simulink model "UAVIntegratedNavigationSystem"  (R2020b)
settings: Solver=FixedStepAuto  StartTime=0.0  StopTime=TFinal  FixedStep=IMUtime  RelTol=1e-3
values from neighbouring files (symbols this model uses):
  AIONtime = 1    [ModelSettings.m]
  BiasAccel = 9.81E-4    (= 0.000981)    [ModelSettings.m]
  BiasGyro = 2.424068405548E-4    (= 0.000242406840555)    [ModelSettings.m]
  CorrTimeOrientationGNSS = 1    [ModelSettings.m]
  CorrTimePositionGNSS = 1    [ModelSettings.m]
  CorrTimeVelocityGNSS = 1    [ModelSettings.m]
  delay = 1.5    [ModelSettings.m]
  e = 0.081819106    [ModelSettings.m]
  g0 = 9.780327    [ModelSettings.m]
  GNSStime = 0.2    [ModelSettings.m]
  H0 = 0.1    [ModelSettings.m]
  IMUtime = 0.01    [ModelSettings.m]
  indUAV = 2    [ModelSettings.m]
  LambdaInit = 0.6555    [ModelSettings.m]
  mass = 0.7    [ModelSettings.m]
  N = 100    [ModelSettings.m]
  PhiInit = 0.968    [ModelSettings.m]
  PitchDown = -PitchUp    (= -0.1)    [ModelSettings.m]
  PitchUp = 0.1    [ModelSettings.m]
  Ra = 6378.245    [ModelSettings.m]
  RollDown = -RollUp    (= -0.1)    [ModelSettings.m]
  RollUp = 0.1    [ModelSettings.m]
  SigmaAccel = 9.81E-4    (= 0.000981)    [ModelSettings.m]
  SigmaAION = 30    [ModelSettings.m]
  SigmaAltitudeGNSS = 3    [ModelSettings.m]
  SigmaGyro = 2.666475246102E-6    (= 2.6664752461e-06)    [ModelSettings.m]
  SigmaLaser = 5    [ModelSettings.m]
  SigmaOrientationGNSS = 0.00349    [ModelSettings.m]
  SigmaPositionGNSS = 1.5    [ModelSettings.m]
  SigmaVelocityGNSS = 0.03    [ModelSettings.m]
  SigmaVelocityUpGNSS = 0.03    [ModelSettings.m]
  U1down = 0    [ModelSettings.m]
  U1up = 4 * ForceCoeff * OmegaMax^2    (= 9.9858124)    [ModelSettings.m]
  U2down = -U2up    (= -2.4964531)    [ModelSettings.m]
  U2up = ForceCoeff * OmegaMax^2    (= 2.4964531)    [ModelSettings.m]
  U3down = -U3up    (= -2.4964531)    [ModelSettings.m]
  U3up = ForceCoeff * OmegaMax^2    (= 2.4964531)    [ModelSettings.m]
  U4down = -U4up    (= -0.2494604)    [ModelSettings.m]
  U4up = 2 * DragCoeff * OmegaMax^2    (= 0.2494604)    [ModelSettings.m]
  WEarth = 7.2921158553E-5    (= 7.2921158553e-05)    [ModelSettings.m]
undefined symbols (not defined in the file or in its folder): deg, Newton, rad, Raphson, s
libraries: simulink x11, sharedtransform x7, pid_lib x6, aerolibconvert2 x4, sharedutil x4
(part 3 of 5)

== system UAVIntegratedNavigationSystem/Subsystem1/Функционирование приемника ГНСС/If Action Subsystem4 ==
  Action Port : ActionPort  ActionPortLabel=if(u1 == -1)
  Bus Creator : BusCreator  Inputs=3
  Mux1 : Mux  Inputs=3
  Mux2 : Mux  Inputs=3
  Mux3 : Mux  Inputs=3
  NaN{,1..8} (9 alike) : Constant  Value=NaN  OutDataTypeStr=Inherit: Inherit via back propagation
  Out1 : Outport
  wires:
  NaN5/1 -> Mux2/3  "<VelZ>"
  NaN1/1 -> Mux1/2  "<Y>"
  NaN4/1 -> Mux2/2  "<VelY>"
  Mux1/1 -> Bus Creator/1
  NaN3/1 -> Mux2/1  "<VelX>"
  NaN/1 -> Mux1/1  "<X>"
  Mux2/1 -> Bus Creator/2
  NaN6/1 -> Mux3/1  "<Roll>"
  NaN2/1 -> Mux1/3  "<Z>"
  Mux3/1 -> Bus Creator/3
  NaN8/1 -> Mux3/2  "<Psi>"
  NaN7/1 -> Mux3/3  "<Pitch>"
  Bus Creator/1 -> Out1/1

== system UAVIntegratedNavigationSystem/Subsystem1/Функционирование приемника ГНСС/If Action Subsystem5 ==
  In1 : Inport
  Action Port : ActionPort  ActionPortLabel=else
  Out1 : Outport
  wires:
  In1/1 -> Out1/1

== system UAVIntegratedNavigationSystem/Алгоритм ИНС /Алгоритм Навигации/Координаты БПЛА (Географ. СК) ==
  Velocity : Inport
  R : Inport  Port=2
  "Север(0), Восток(0)" : Inport  Port=3
  Demux : Demux  Outputs=2
  Demux1 : Demux  Outputs=3
  Demux2 : Demux  Outputs=2
  Integrator : Integrator  InitialCondition=PhiInit
  Integrator1 : Integrator  InitialConditionSource=external
  Integrator2 : Integrator
  Integrator3 : Integrator  InitialConditionSource=external
  Mux : Mux
  Terminator : Terminator
  dPhi/dt : Product  Inputs=*/
  "Coord, phi" : Outport
  wires:
  R/1 -> Demux/1
  dPhi/dt/1 -> Integrator/1
  Demux/1 -> dPhi/dt/2
  Velocity/1 -> Demux1/1
  Demux1/1 -> dPhi/dt/1, Integrator1/1
  Mux/1 -> "Coord, phi"/1
  Demux/2 -> Terminator/1
  Integrator1/1 -> Mux/1
  Integrator2/1 -> Mux/2
  Integrator3/1 -> Mux/3
  Demux1/2 -> Integrator2/1
  Demux1/3 -> Integrator3/1
  Integrator/1 -> Mux/4
  "Север(0), Восток(0)"/1 -> Demux2/1
  Demux2/1 -> Integrator1/2
  Demux2/2 -> Integrator3/2

== system UAVIntegratedNavigationSystem/Алгоритм ИНС /Алгоритм Навигации/Радиус - вектор точки местоположения Ц.М. БПЛА (phi) ==
  Phi : Inport
  Add2 : Sum  Inputs=+-
  Add3 : Sum  Inputs=+-
  Add4 : Sum
  Add5 : Sum
  Constant2 : Constant  Value=Ra
  Constant3 : Constant  Value=H0
  Constant4 : Constant
  Constant5 : Constant  Value=1.5
  Divide : Product  Inputs=*/
  Divide1 : Product  Inputs=*/
  Mux : Mux  Inputs=2
  Power : Math  Operator=pow  SaturateOnIntegerOverflow=on
  Product1 : Product
  Product2 : Product
  Sin1 : Trigonometry
  Sqrt : Sqrt  SaturateOnIntegerOverflow=on
  Square2 : Math  Operator=square  SaturateOnIntegerOverflow=on
  Square3 : Math  Operator=square  SaturateOnIntegerOverflow=on
  e1 : Constant  Value=e
  "km -> m" : Gain  Gain=1000
  "km -> m 1" : Gain  Gain=1000
  "R, м" : Outport
  wires:
  Phi/1 -> Sin1/1
  Constant2/1 -> "km -> m"/1
  Constant3/1 -> "km -> m 1"/1
  e1/1 -> Square2/1
  Square2/1 -> Product2/1, Add2/2
  Constant4/1 -> Add2/1, Add3/1
  "km -> m"/1 -> Product1/1, Divide1/1
  Add2/1 -> Product1/2
  Sin1/1 -> Square3/1
  Square3/1 -> Product2/2
  Product2/1 -> Add3/2
  Product1/1 -> Divide/1
  Divide/1 -> Add4/1
  "km -> m 1"/1 -> Add5/1, Add4/2
  Add4/1 -> Mux/1  "R1"
  Add3/1 -> Power/1, Sqrt/1
  Power/1 -> Divide/2
  Constant5/1 -> Power/2
  Mux/1 -> "R, м"/1
  Sqrt/1 -> Divide1/2
  Divide1/1 -> Add5/2
  Add5/1 -> Mux/2  "R2"

== system UAVIntegratedNavigationSystem/Алгоритм ИНС /Алгоритм Навигации/Скорости БПЛА (Географ. СК) ==
  AccX : Inport
  AccY : Inport  Port=2
  AccZ : Inport  Port=3
  R : Inport  Port=4
  phi : Inport  Port=5
  Integrator : Integrator
  Integrator1 : Integrator
  Integrator2 : Integrator
  Mux : Mux  Inputs=3
  dVx / dt : Subsystem
  dVy / dt : Subsystem
  dVz / dt : Subsystem
  Velocity : Outport
  wires:
  Integrator/1 -> dVz / dt/5(Vx), dVy / dt/4(Vx), dVx / dt/5(Vx), Mux/1
  Integrator1/1 -> dVz / dt/3(Vy), dVx / dt/3(Vy), Mux/2
  Integrator2/1 -> Mux/3, dVz / dt/4(Vz), dVx / dt/4(Vz), dVy / dt/3(Vz)
  AccX/1 -> dVx / dt/1(AccX)
  R/1 -> dVz / dt/2(R), dVy / dt/2(R), dVx / dt/2(R)
  dVx / dt/1(dVx/dt) -> Integrator/1
  AccY/1 -> dVy / dt/1(AccY)
  dVy / dt/1(dVy/dt) -> Integrator1/1
  AccZ/1 -> dVz / dt/1(AccZ)
  dVz / dt/1(dVz/dt) -> Integrator2/1
  Mux/1 -> Velocity/1
  phi/1 -> dVx / dt/6(phi), dVy / dt/5(phi), dVz / dt/6(phi)

== system UAVIntegratedNavigationSystem/Алгоритм ИНС /Алгоритм Навигации/Угловая скорость вращения трехгранника ==
  Velocity : Inport
  R : Inport  Port=2
  phi : Inport  Port=3
  Add : Sum
  Constant : Constant  Value=0
  Cos : Trigonometry  Operator=cos
  Demux2 : Demux  Outputs=3
  Demux3 : Demux  Outputs=2
  Divide : Product  Inputs=*/
  Divide1 : Product  Inputs=*/
  Divide2 : Product  Inputs=*/
  Gain : Gain  Gain=-1
  Mux : Mux  Inputs=3
  Mux1 : Mux  Inputs=3
  Sin : Trigonometry
  Terminator3 : Terminator
  WEarth : Gain  Gain=WEarth
  WEarth1 : Gain  Gain=WEarth
  OmegaG : Outport
  wires:
  Demux2/3 -> Divide/1, Divide1/1
  phi/1 -> Sin/1, Cos/1
  WEarth1/1 -> Mux1/2
  Cos/1 -> WEarth/1
  Divide/1 -> Mux/1
  Sin/1 -> WEarth1/1
  WEarth/1 -> Mux1/1
  R/1 -> Demux3/1
  Constant/1 -> Mux1/3
  Demux3/2 -> Divide1/2
  Mux/1 -> Add/2
  Demux2/1 -> Gain/1
  Add/1 -> OmegaG/1
  Demux2/2 -> Terminator3/1
  Demux3/1 -> Divide/2, Divide2/2
  Divide2/1 -> Mux/3
  Divide1/1 -> Mux/2
  Mux1/1 -> Add/1
  Gain/1 -> Divide2/1
  Velocity/1 -> Demux2/1

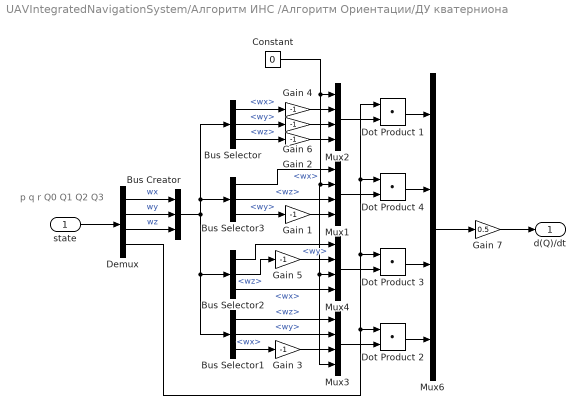
== system UAVIntegratedNavigationSystem/Алгоритм ИНС /Алгоритм Ориентации/ДУ кватерниона ==
  note: p q r Q0 Q1 Q2 Q3
  state : Inport
  Bus Creator : BusCreator  Inputs=3
  Bus Selector : BusSelector  OutputSignals=wx,wy,wz
  Bus Selector1 : BusSelector  OutputSignals=wz,wy,wx
  Bus Selector2 : BusSelector  OutputSignals=wy,wz,wx
  Bus Selector3 : BusSelector  OutputSignals=wx,wz,wy
  Constant : Constant  Value=0
  Demux : Demux  Outputs=[1 1 1 4]
      settings: DisplayOption=none
  Dot Product {1..4} (4 alike) : DotProduct  InputSameDT=on  OutDataTypeStr=Inherit: Inherit via internal rule
  Gain {1..6} (6 alike) : Gain  Gain=-1  SaturateOnIntegerOverflow=on  OutDataTypeStr=Inherit: Same as input  ParamDataTypeStr=Inherit: Same as input
  Gain 7 : Gain  Gain=0.5  SaturateOnIntegerOverflow=on  OutDataTypeStr=Inherit: Same as input  ParamDataTypeStr=Inherit: Same as input
  Mux{1..4,6} (5 alike) : Mux
  d(Q)/dt : Outport
  wires:
  Mux6/1 -> Gain 7/1
  state/1 -> Demux/1
  Gain 2/1 -> Mux2/4
  Bus Selector/1 -> Gain 4/1  "<wx>"
  Mux2/1 -> Dot Product 1/2
  Mux3/1 -> Dot Product 2/2
  Mux4/1 -> Dot Product 3/2
  Demux/1 -> Bus Creator/1  "wx"
  Demux/2 -> Bus Creator/2  "wy"
  Demux/3 -> Bus Creator/3  "wz"
  Gain 5/1 -> Mux4/2
  Gain 3/1 -> Mux3/3
  Mux1/1 -> Dot Product 4/2
  Bus Creator/1 -> Bus Selector2/1, Bus Selector1/1, Bus Selector/1, Bus Selector3/1
  Constant/1 -> Mux2/1, Mux1/2, Mux3/4, Mux4/3
  Bus Selector3/3 -> Gain 1/1  "<wy>"
  Gain 4/1 -> Mux2/2
  Gain 6/1 -> Mux2/3
  Bus Selector/2 -> Gain 6/1  "<wy>"
  Bus Selector/3 -> Gain 2/1  "<wz>"
  Dot Product 2/1 -> Mux6/4
  Dot Product 3/1 -> Mux6/3
  Dot Product 4/1 -> Mux6/2
  Dot Product 1/1 -> Mux6/1
  Demux/4 -> Dot Product 3/1, Dot Product 4/1, Dot Product 1/1, Dot Product 2/1
  Gain 7/1 -> d(Q)/dt/1
  Bus Selector3/1 -> Mux1/1  "<wx>"
  Bus Selector3/2 -> Mux1/3  "<wz>"
  Gain 1/1 -> Mux1/4
  Bus Selector1/3 -> Gain 3/1  "<wx>"
  Bus Selector1/2 -> Mux3/2  "<wy>"
  Bus Selector1/1 -> Mux3/1  "<wz>"
  Bus Selector2/1 -> Mux4/1  "<wy>"
  Bus Selector2/2 -> Gain 5/1  "<wz>"
  Bus Selector2/3 -> Mux4/4  "<wx>"

== system UAVIntegratedNavigationSystem/Алгоритм ИНС /Алгоритм Ориентации/Нормирование кватерниона ==
  q : Inport  PortDimensions=4
  Product : Product  Inputs=*/  InputSameDT=on  RndMeth=Zero  SaturateOnIntegerOverflow=on  OutDataTypeStr=Inherit: Same as first input
  Square : Math  Operator=square  SignedPower=on  SaturateOnIntegerOverflow=on
  Square Root : Sqrt  Operator=signedSqrt  AlgorithmType=Newton-Raphson  SaturateOnIntegerOverflow=on
  Sum : Sum  Inputs=1  InputSameDT=on  SaturateOnIntegerOverflow=on  OutDataTypeStr=Inherit: Same as first input
  qnorm : Outport  PortDimensions=4
  wires:
  Product/1 -> qnorm/1
  Square Root/1 -> Product/2
  Square/1 -> Sum/1
  Sum/1 -> Square Root/1
  q/1 -> Product/1, Square/1

== system UAVIntegratedNavigationSystem/Алгоритм ИНС (коррекия БЧЭ)/Алгоритм Навигации/Координаты БПЛА (Географ. СК) ==
  Velocity : Inport
  R : Inport  Port=2
  "Север(0), Восток(0)" : Inport  Port=3
  Demux : Demux  Outputs=2
  Demux1 : Demux  Outputs=3
  Demux2 : Demux  Outputs=2
  Integrator : Integrator  InitialCondition=PhiInit
  Integrator1 : Integrator  InitialConditionSource=external
  Integrator2 : Integrator
  Integrator3 : Integrator  InitialConditionSource=external
  Mux : Mux
  Terminator : Terminator
  dPhi/dt : Product  Inputs=*/
  "Coord, phi" : Outport
  wires:
  R/1 -> Demux/1
  dPhi/dt/1 -> Integrator/1
  Demux/1 -> dPhi/dt/2
  Velocity/1 -> Demux1/1
  Demux1/1 -> dPhi/dt/1, Integrator1/1
  Mux/1 -> "Coord, phi"/1
  Demux/2 -> Terminator/1
  Integrator1/1 -> Mux/1
  Integrator2/1 -> Mux/2
  Integrator3/1 -> Mux/3
  Demux1/2 -> Integrator2/1
  Demux1/3 -> Integrator3/1
  Integrator/1 -> Mux/4
  "Север(0), Восток(0)"/1 -> Demux2/1
  Demux2/1 -> Integrator1/2
  Demux2/2 -> Integrator3/2

== system UAVIntegratedNavigationSystem/Алгоритм ИНС (коррекия БЧЭ)/Алгоритм Навигации/Радиус - вектор точки местоположения Ц.М. БПЛА (phi) ==
  Phi : Inport
  Add2 : Sum  Inputs=+-
  Add3 : Sum  Inputs=+-
  Add4 : Sum
  Add5 : Sum
  Constant2 : Constant  Value=Ra
  Constant3 : Constant  Value=H0
  Constant4 : Constant
  Constant5 : Constant  Value=1.5
  Divide : Product  Inputs=*/
  Divide1 : Product  Inputs=*/
  Mux : Mux  Inputs=2
  Power : Math  Operator=pow  SaturateOnIntegerOverflow=on
  Product1 : Product
  Product2 : Product
  Sin1 : Trigonometry
  Sqrt : Sqrt  SaturateOnIntegerOverflow=on
  Square2 : Math  Operator=square  SaturateOnIntegerOverflow=on
  Square3 : Math  Operator=square  SaturateOnIntegerOverflow=on
  e1 : Constant  Value=e
  "km -> m" : Gain  Gain=1000
  "km -> m 1" : Gain  Gain=1000
  "R, м" : Outport
  wires:
  Phi/1 -> Sin1/1
  Constant2/1 -> "km -> m"/1
  Constant3/1 -> "km -> m 1"/1
  e1/1 -> Square2/1
  Square2/1 -> Product2/1, Add2/2
  Constant4/1 -> Add2/1, Add3/1
  "km -> m"/1 -> Product1/1, Divide1/1
  Add2/1 -> Product1/2
  Sin1/1 -> Square3/1
  Square3/1 -> Product2/2
  Product2/1 -> Add3/2
  Product1/1 -> Divide/1
  Divide/1 -> Add4/1
  "km -> m 1"/1 -> Add5/1, Add4/2
  Add4/1 -> Mux/1  "R1"
  Add3/1 -> Power/1, Sqrt/1
  Power/1 -> Divide/2
  Constant5/1 -> Power/2
  Mux/1 -> "R, м"/1
  Sqrt/1 -> Divide1/2
  Divide1/1 -> Add5/2
  Add5/1 -> Mux/2  "R2"

== system UAVIntegratedNavigationSystem/Алгоритм ИНС (коррекия БЧЭ)/Алгоритм Навигации/Скорости БПЛА (Географ. СК) ==
  AccX : Inport
  AccY : Inport  Port=2
  AccZ : Inport  Port=3
  R : Inport  Port=4
  phi : Inport  Port=5
  Integrator : Integrator
  Integrator1 : Integrator
  Integrator2 : Integrator
  Mux : Mux  Inputs=3
  dVx / dt : Subsystem
  dVy / dt : Subsystem
  dVz / dt : Subsystem
  Velocity : Outport
  wires:
  Integrator/1 -> dVz / dt/5(Vx), dVy / dt/4(Vx), dVx / dt/5(Vx), Mux/1
  Integrator1/1 -> dVz / dt/3(Vy), dVx / dt/3(Vy), Mux/2
  Integrator2/1 -> Mux/3, dVz / dt/4(Vz), dVx / dt/4(Vz), dVy / dt/3(Vz)
  AccX/1 -> dVx / dt/1(AccX)
  R/1 -> dVz / dt/2(R), dVy / dt/2(R), dVx / dt/2(R)
  dVx / dt/1(dVx/dt) -> Integrator/1
  AccY/1 -> dVy / dt/1(AccY)
  dVy / dt/1(dVy/dt) -> Integrator1/1
  AccZ/1 -> dVz / dt/1(AccZ)
  dVz / dt/1(dVz/dt) -> Integrator2/1
  Mux/1 -> Velocity/1
  phi/1 -> dVx / dt/6(phi), dVy / dt/5(phi), dVz / dt/6(phi)

== system UAVIntegratedNavigationSystem/Алгоритм ИНС (коррекия БЧЭ)/Алгоритм Навигации/Угловая скорость вращения трехгранника ==
  Velocity : Inport
  R : Inport  Port=2
  phi : Inport  Port=3
  Add : Sum
  Constant : Constant  Value=0
  Cos : Trigonometry  Operator=cos
  Demux2 : Demux  Outputs=3
  Demux3 : Demux  Outputs=2
  Divide : Product  Inputs=*/
  Divide1 : Product  Inputs=*/
  Divide2 : Product  Inputs=*/
  Gain : Gain  Gain=-1
  Mux : Mux  Inputs=3
  Mux1 : Mux  Inputs=3
  Sin : Trigonometry
  Terminator3 : Terminator
  WEarth : Gain  Gain=WEarth
  WEarth1 : Gain  Gain=WEarth
  OmegaG : Outport
  wires:
  Demux2/3 -> Divide/1, Divide1/1
  phi/1 -> Sin/1, Cos/1
  WEarth1/1 -> Mux1/2
  Cos/1 -> WEarth/1
  Divide/1 -> Mux/1
  Sin/1 -> WEarth1/1
  WEarth/1 -> Mux1/1
  R/1 -> Demux3/1
  Constant/1 -> Mux1/3
  Demux3/2 -> Divide1/2
  Mux/1 -> Add/2
  Demux2/1 -> Gain/1
  Add/1 -> OmegaG/1
  Demux2/2 -> Terminator3/1
  Demux3/1 -> Divide/2, Divide2/2
  Divide2/1 -> Mux/3
  Divide1/1 -> Mux/2
  Mux1/1 -> Add/1
  Gain/1 -> Divide2/1
  Velocity/1 -> Demux2/1

== system UAVIntegratedNavigationSystem/Алгоритм ИНС (коррекия БЧЭ)/Алгоритм Ориентации/ДУ кватерниона ==
  note: p q r Q0 Q1 Q2 Q3
  state : Inport
  Bus Creator : BusCreator  Inputs=3
  Bus Selector : BusSelector  OutputSignals=wx,wy,wz
  Bus Selector1 : BusSelector  OutputSignals=wz,wy,wx
  Bus Selector2 : BusSelector  OutputSignals=wy,wz,wx
  Bus Selector3 : BusSelector  OutputSignals=wx,wz,wy
  Constant : Constant  Value=0
  Demux : Demux  Outputs=[1 1 1 4]
      settings: DisplayOption=none
  Dot Product {1..4} (4 alike) : DotProduct  InputSameDT=on  OutDataTypeStr=Inherit: Inherit via internal rule
  Gain {1..6} (6 alike) : Gain  Gain=-1  SaturateOnIntegerOverflow=on  OutDataTypeStr=Inherit: Same as input  ParamDataTypeStr=Inherit: Same as input
  Gain 7 : Gain  Gain=0.5  SaturateOnIntegerOverflow=on  OutDataTypeStr=Inherit: Same as input  ParamDataTypeStr=Inherit: Same as input
  Mux{1..4,6} (5 alike) : Mux
  d(Q)/dt : Outport
  wires:
  Mux6/1 -> Gain 7/1
  state/1 -> Demux/1
  Gain 2/1 -> Mux2/4
  Bus Selector/1 -> Gain 4/1  "<wx>"
  Mux2/1 -> Dot Product 1/2
  Mux3/1 -> Dot Product 2/2
  Mux4/1 -> Dot Product 3/2
  Demux/1 -> Bus Creator/1  "wx"
  Demux/2 -> Bus Creator/2  "wy"
  Demux/3 -> Bus Creator/3  "wz"
  Gain 5/1 -> Mux4/2
  Gain 3/1 -> Mux3/3
  Mux1/1 -> Dot Product 4/2
  Bus Creator/1 -> Bus Selector2/1, Bus Selector1/1, Bus Selector/1, Bus Selector3/1
  Constant/1 -> Mux2/1, Mux1/2, Mux3/4, Mux4/3
  Bus Selector3/3 -> Gain 1/1  "<wy>"
  Gain 4/1 -> Mux2/2
  Gain 6/1 -> Mux2/3
  Bus Selector/2 -> Gain 6/1  "<wy>"
  Bus Selector/3 -> Gain 2/1  "<wz>"
  Dot Product 2/1 -> Mux6/4
  Dot Product 3/1 -> Mux6/3
  Dot Product 4/1 -> Mux6/2
  Dot Product 1/1 -> Mux6/1
  Demux/4 -> Dot Product 3/1, Dot Product 4/1, Dot Product 1/1, Dot Product 2/1
  Gain 7/1 -> d(Q)/dt/1
  Bus Selector3/1 -> Mux1/1  "<wx>"
  Bus Selector3/2 -> Mux1/3  "<wz>"
  Gain 1/1 -> Mux1/4
  Bus Selector1/3 -> Gain 3/1  "<wx>"
  Bus Selector1/2 -> Mux3/2  "<wy>"
  Bus Selector1/1 -> Mux3/1  "<wz>"
  Bus Selector2/1 -> Mux4/1  "<wy>"
  Bus Selector2/2 -> Gain 5/1  "<wz>"
  Bus Selector2/3 -> Mux4/4  "<wx>"

== system UAVIntegratedNavigationSystem/Алгоритм ИНС (коррекия БЧЭ)/Алгоритм Ориентации/Нормирование кватерниона ==
  q : Inport  PortDimensions=4
  Product : Product  Inputs=*/  InputSameDT=on  RndMeth=Zero  SaturateOnIntegerOverflow=on  OutDataTypeStr=Inherit: Same as first input
  Square : Math  Operator=square  SignedPower=on  SaturateOnIntegerOverflow=on
  Square Root : Sqrt  Operator=signedSqrt  AlgorithmType=Newton-Raphson  SaturateOnIntegerOverflow=on
  Sum : Sum  Inputs=1  InputSameDT=on  SaturateOnIntegerOverflow=on  OutDataTypeStr=Inherit: Same as first input
  qnorm : Outport  PortDimensions=4
  wires:
  Product/1 -> qnorm/1
  Square Root/1 -> Product/2
  Square/1 -> Sum/1
  Sum/1 -> Square Root/1
  q/1 -> Product/1, Square/1

== system UAVIntegratedNavigationSystem/Блок модели динамики квадрокоптера + САУ/Полетный контроллер/Ограничение управляющих сил ==
  U1* : Inport
  U2* : Inport  Port=2
  U3* : Inport  Port=3
  U4* : Inport  Port=4
  Limit U1 : Saturate  UpperLimit=U1up  LowerLimit=U1down
  Limit U2 : Saturate  UpperLimit=U2up  LowerLimit=U2down
  Limit U3 : Saturate  UpperLimit=U3up  LowerLimit=U3down
  Limit U4 : Saturate  UpperLimit=U4up  LowerLimit=U4down
  U1 : Outport
  U2 : Outport  Port=2
  U3 : Outport  Port=3
  U4 : Outport  Port=4
  wires:
  Limit U2/1 -> U2/1
  U2*/1 -> Limit U2/1
  U1*/1 -> Limit U1/1
  Limit U1/1 -> U1/1
  U4*/1 -> Limit U4/1
  Limit U4/1 -> U4/1
  Limit U3/1 -> U3/1
  U3*/1 -> Limit U3/1

== system UAVIntegratedNavigationSystem/Блок модели динамики квадрокоптера + САУ/Полетный контроллер/Угловая стабилизация ==
  Roll* : Inport
  Roll : Inport  Port=2
  Pitch* : Inport  Port=3
  Pitch : Inport  Port=4
  Psi* : Inport  Port=5
  Psi : Inport  Port=6
  RollPID : Inport  Port=7
  PitchPID : Inport  Port=8
  PsiPID : Inport  Port=9
  Constant : Constant  Value=N
  Demux : Demux  Outputs=3
  Demux1 : Demux  Outputs=3
  Demux2 : Demux  Outputs=3
  PID Pitch : pid_lib/PID Controller  Controller=PID  Form=Parallel  TimeDomain=Continuous-time  UseExternalTs=off  SampleTime=-1  IntegratorMethod=Forward Euler  FilterMethod=Forward Euler  ControllerParametersSource=external  P=1  I=0  D=0  UseFilter=on  N=100  TunerSelectOption=Transfer Function Based (PID Tuner App)  InitialConditionSource=internal  InitialConditionForIntegrator=0  InitialConditionForFilter=0  DifferentiatorICPrevScaledInput=0  ExternalReset=none  TrackingMode=off  Kt=1  LimitOutput=off  SatLimitsSource=internal  UpperSaturationLimit=inf  LowerSaturationLimit=-inf  LinearizeAsGain=on  AntiWindupMode=none  Kb=1  POutMin=[]  POutMax=[]  IOutMin=[]  IOutMax=[]  DOutMin=[]  DOutMax=[]  NOutMin=[]  NOutMax=[]  SumOutMin=[]  SumOutMax=[]  SaturationOutMin=[]  SaturationOutMax=[]  PParamMin=[]  PParamMax=[]  IParamMin=[]  IParamMax=[]  DParamMin=[]  DParamMax=[]  NParamMin=[]  NParamMax=[]  KbParamMin=[]  KbParamMax=[]  KtParamMin=[]  KtParamMax=[]  KbOutMin=[]  KbOutMax=[]  KtOutMin=[]  KtOutMax=[]  IntegratorOutMin=[]  IntegratorOutMax=[]  FilterOutMin=[]  FilterOutMax=[]  SumI1OutMin=[]  SumI1OutMax=[]  SumI2OutMin=[]  SumI2OutMax=[]  SumI3OutMin=[]  SumI3OutMax=[]  SumI4OutMin=[]  SumI4OutMax=[]  SumDOutMin=[]  SumDOutMax=[]  DifferentiatorOutMin=[]  DifferentiatorOutMax=[]  FilterDiffOutCoefMin=[]  FilterDiffOutCoefMax=[]  ReciprocalOutMin=[]  ReciprocalOutMax=[]  SumDenOutMin=[]  SumDenOutMax=[]  SumNumOutMin=[]  SumNumOutMax=[]  DivideOutMin=[]  DivideOutMax=[]  UdiffTsProdOutMin=[]  UdiffTsProdOutMax=[]  NTsProdOutMin=[]  NTsProdOutMax=[]  UintegralTsProdOutMin=[]  UintegralTsProdOutMax=[]  UngainTsProdOutMin=[]  UngainTsProdOutMax=[]  IntegratorContinuousStateAttributes=''  IntegratorStateMustResolveToSignalObject=off  IntegratorRTWStateStorageClass=Auto  FilterContinuousStateAttributes=''  FilterStateMustResolveToSignalObject=off  FilterRTWStateStorageClass=Auto  ParallelPVariant=ExternalParameters  IdealPVariant=Disabled  IVariant=ExternalParameters  DVariant=ExternalParameters  IntegratorVariant=Continuous  SatVariant=Disabled  AWVariant=Passthrough  PCopyVariant=Disabled  TRVariant=Disabled  FdbkBlocksVariant=Forward  IdealPFdbkVariant=Disabled  SatFdbkVariant=Disabled  DerivativeFilterVariant=ContFilter  NVariant=ExternalParameters  NCopyVariant=Disabled  FilterICVariant=InternalICsFilter  IntegratorICVariant=InternalICs  ExternalResetVariant=Disabled  TRSumVariant=Passthrough  SumFdbkVariant=Disabled  SumVariant=Sum_PID  TsampFilterVariant=InternalTs  TsampNgainVariant=Passthrough  TsampIntegralVariant=Passthrough  ExternalSaturationOutDataTypeStr=Inherit: Same as second input
  PID Psi : pid_lib/PID Controller  Controller=PID  Form=Parallel  TimeDomain=Continuous-time  UseExternalTs=off  SampleTime=-1  IntegratorMethod=Forward Euler  FilterMethod=Forward Euler  ControllerParametersSource=external  P=1  I=0  D=0  UseFilter=on  N=100  TunerSelectOption=Transfer Function Based (PID Tuner App)  InitialConditionSource=internal  InitialConditionForIntegrator=0  InitialConditionForFilter=0  DifferentiatorICPrevScaledInput=0  ExternalReset=none  TrackingMode=off  Kt=1  LimitOutput=off  SatLimitsSource=internal  UpperSaturationLimit=inf  LowerSaturationLimit=-inf  LinearizeAsGain=on  AntiWindupMode=none  Kb=1  POutMin=[]  POutMax=[]  IOutMin=[]  IOutMax=[]  DOutMin=[]  DOutMax=[]  NOutMin=[]  NOutMax=[]  SumOutMin=[]  SumOutMax=[]  SaturationOutMin=[]  SaturationOutMax=[]  PParamMin=[]  PParamMax=[]  IParamMin=[]  IParamMax=[]  DParamMin=[]  DParamMax=[]  NParamMin=[]  NParamMax=[]  KbParamMin=[]  KbParamMax=[]  KtParamMin=[]  KtParamMax=[]  KbOutMin=[]  KbOutMax=[]  KtOutMin=[]  KtOutMax=[]  IntegratorOutMin=[]  IntegratorOutMax=[]  FilterOutMin=[]  FilterOutMax=[]  SumI1OutMin=[]  SumI1OutMax=[]  SumI2OutMin=[]  SumI2OutMax=[]  SumI3OutMin=[]  SumI3OutMax=[]  SumI4OutMin=[]  SumI4OutMax=[]  SumDOutMin=[]  SumDOutMax=[]  DifferentiatorOutMin=[]  DifferentiatorOutMax=[]  FilterDiffOutCoefMin=[]  FilterDiffOutCoefMax=[]  ReciprocalOutMin=[]  ReciprocalOutMax=[]  SumDenOutMin=[]  SumDenOutMax=[]  SumNumOutMin=[]  SumNumOutMax=[]  DivideOutMin=[]  DivideOutMax=[]  UdiffTsProdOutMin=[]  UdiffTsProdOutMax=[]  NTsProdOutMin=[]  NTsProdOutMax=[]  UintegralTsProdOutMin=[]  UintegralTsProdOutMax=[]  UngainTsProdOutMin=[]  UngainTsProdOutMax=[]  IntegratorContinuousStateAttributes=''  IntegratorStateMustResolveToSignalObject=off  IntegratorRTWStateStorageClass=Auto  FilterContinuousStateAttributes=''  FilterStateMustResolveToSignalObject=off  FilterRTWStateStorageClass=Auto  ParallelPVariant=ExternalParameters  IdealPVariant=Disabled  IVariant=ExternalParameters  DVariant=ExternalParameters  IntegratorVariant=Continuous  SatVariant=Disabled  AWVariant=Passthrough  PCopyVariant=Disabled  TRVariant=Disabled  FdbkBlocksVariant=Forward  IdealPFdbkVariant=Disabled  SatFdbkVariant=Disabled  DerivativeFilterVariant=ContFilter  NVariant=ExternalParameters  NCopyVariant=Disabled  FilterICVariant=InternalICsFilter  IntegratorICVariant=InternalICs  ExternalResetVariant=Disabled  TRSumVariant=Passthrough  SumFdbkVariant=Disabled  SumVariant=Sum_PID  TsampFilterVariant=InternalTs  TsampNgainVariant=Passthrough  TsampIntegralVariant=Passthrough  ExternalSaturationOutDataTypeStr=Inherit: Same as second input
  PID Roll : pid_lib/PID Controller  Controller=PID  Form=Parallel  TimeDomain=Continuous-time  UseExternalTs=off  SampleTime=-1  IntegratorMethod=Forward Euler  FilterMethod=Forward Euler  ControllerParametersSource=external  P=1  I=0  D=0  UseFilter=on  N=100  TunerSelectOption=Transfer Function Based (PID Tuner App)  InitialConditionSource=internal  InitialConditionForIntegrator=0  InitialConditionForFilter=0  DifferentiatorICPrevScaledInput=0  ExternalReset=none  TrackingMode=off  Kt=1  LimitOutput=off  SatLimitsSource=internal  UpperSaturationLimit=inf  LowerSaturationLimit=-inf  LinearizeAsGain=on  AntiWindupMode=none  Kb=1  POutMin=[]  POutMax=[]  IOutMin=[]  IOutMax=[]  DOutMin=[]  DOutMax=[]  NOutMin=[]  NOutMax=[]  SumOutMin=[]  SumOutMax=[]  SaturationOutMin=[]  SaturationOutMax=[]  PParamMin=[]  PParamMax=[]  IParamMin=[]  IParamMax=[]  DParamMin=[]  DParamMax=[]  NParamMin=[]  NParamMax=[]  KbParamMin=[]  KbParamMax=[]  KtParamMin=[]  KtParamMax=[]  KbOutMin=[]  KbOutMax=[]  KtOutMin=[]  KtOutMax=[]  IntegratorOutMin=[]  IntegratorOutMax=[]  FilterOutMin=[]  FilterOutMax=[]  SumI1OutMin=[]  SumI1OutMax=[]  SumI2OutMin=[]  SumI2OutMax=[]  SumI3OutMin=[]  SumI3OutMax=[]  SumI4OutMin=[]  SumI4OutMax=[]  SumDOutMin=[]  SumDOutMax=[]  DifferentiatorOutMin=[]  DifferentiatorOutMax=[]  FilterDiffOutCoefMin=[]  FilterDiffOutCoefMax=[]  ReciprocalOutMin=[]  ReciprocalOutMax=[]  SumDenOutMin=[]  SumDenOutMax=[]  SumNumOutMin=[]  SumNumOutMax=[]  DivideOutMin=[]  DivideOutMax=[]  UdiffTsProdOutMin=[]  UdiffTsProdOutMax=[]  NTsProdOutMin=[]  NTsProdOutMax=[]  UintegralTsProdOutMin=[]  UintegralTsProdOutMax=[]  UngainTsProdOutMin=[]  UngainTsProdOutMax=[]  IntegratorContinuousStateAttributes=''  IntegratorStateMustResolveToSignalObject=off  IntegratorRTWStateStorageClass=Auto  FilterContinuousStateAttributes=''  FilterStateMustResolveToSignalObject=off  FilterRTWStateStorageClass=Auto  ParallelPVariant=ExternalParameters  IdealPVariant=Disabled  IVariant=ExternalParameters  DVariant=ExternalParameters  IntegratorVariant=Continuous  SatVariant=Disabled  AWVariant=Passthrough  PCopyVariant=Disabled  TRVariant=Disabled  FdbkBlocksVariant=Forward  IdealPFdbkVariant=Disabled  SatFdbkVariant=Disabled  DerivativeFilterVariant=ContFilter  NVariant=ExternalParameters  NCopyVariant=Disabled  FilterICVariant=InternalICsFilter  IntegratorICVariant=InternalICs  ExternalResetVariant=Disabled  TRSumVariant=Passthrough  SumFdbkVariant=Disabled  SumVariant=Sum_PID  TsampFilterVariant=InternalTs  TsampNgainVariant=Passthrough  TsampIntegralVariant=Passthrough  ExternalSaturationOutDataTypeStr=Inherit: Same as second input
  Sum1 : Sum  Inputs=|+-
  Sum3 : Sum  Inputs=|+-
  Sum4 : Sum  Inputs=|+-
  U2* : Outport
  U3* : Outport  Port=2
  U4* : Outport  Port=3
  wires:
  Pitch/1 -> Sum4/2
  Psi*/1 -> Sum3/1
  PID Psi/1 -> U4*/1
  Roll/1 -> Sum1/2
  PID Pitch/1 -> U3*/1
  Roll*/1 -> Sum1/1
  Psi/1 -> Sum3/2
  PID Roll/1 -> U2*/1
  Pitch*/1 -> Sum4/1
  Sum1/1 -> PID Roll/1
  Sum4/1 -> PID Pitch/1
  Sum3/1 -> PID Psi/1
  RollPID/1 -> Demux/1
  Demux/3 -> PID Roll/4
  Demux/1 -> PID Roll/2
  Demux/2 -> PID Roll/3
  Constant/1 -> PID Psi/5, PID Pitch/5, PID Roll/5
  Demux1/1 -> PID Pitch/2
  Demux1/2 -> PID Pitch/3
  Demux1/3 -> PID Pitch/4
  PitchPID/1 -> Demux1/1
  Demux2/1 -> PID Psi/2
  Demux2/2 -> PID Psi/3
  Demux2/3 -> PID Psi/4
  PsiPID/1 -> Demux2/1

== system UAVIntegratedNavigationSystem/Блок модели динамики квадрокоптера + САУ/Полетный контроллер/Удержание высоты  ==
  Y* : Inport
  Y : Inport  Port=2
  g : Inport  Port=3
  AltPID : Inport  Port=4
  Add : Sum
  Constant : Constant  Value=N
  Demux : Demux  Outputs=3
  PID Altitude : pid_lib/PID Controller  Controller=PID  Form=Parallel  TimeDomain=Continuous-time  UseExternalTs=off  SampleTime=-1  IntegratorMethod=Forward Euler  FilterMethod=Forward Euler  ControllerParametersSource=external  P=1  I=0  D=0  UseFilter=on  N=100  TunerSelectOption=Transfer Function Based (PID Tuner App)  InitialConditionSource=internal  InitialConditionForIntegrator=0  InitialConditionForFilter=0  DifferentiatorICPrevScaledInput=0  ExternalReset=none  TrackingMode=off  Kt=1  LimitOutput=off  SatLimitsSource=internal  UpperSaturationLimit=inf  LowerSaturationLimit=-inf  LinearizeAsGain=on  AntiWindupMode=none  Kb=1  POutMin=[]  POutMax=[]  IOutMin=[]  IOutMax=[]  DOutMin=[]  DOutMax=[]  NOutMin=[]  NOutMax=[]  SumOutMin=[]  SumOutMax=[]  SaturationOutMin=[]  SaturationOutMax=[]  PParamMin=[]  PParamMax=[]  IParamMin=[]  IParamMax=[]  DParamMin=[]  DParamMax=[]  NParamMin=[]  NParamMax=[]  KbParamMin=[]  KbParamMax=[]  KtParamMin=[]  KtParamMax=[]  KbOutMin=[]  KbOutMax=[]  KtOutMin=[]  KtOutMax=[]  IntegratorOutMin=[]  IntegratorOutMax=[]  FilterOutMin=[]  FilterOutMax=[]  SumI1OutMin=[]  SumI1OutMax=[]  SumI2OutMin=[]  SumI2OutMax=[]  SumI3OutMin=[]  SumI3OutMax=[]  SumI4OutMin=[]  SumI4OutMax=[]  SumDOutMin=[]  SumDOutMax=[]  DifferentiatorOutMin=[]  DifferentiatorOutMax=[]  FilterDiffOutCoefMin=[]  FilterDiffOutCoefMax=[]  ReciprocalOutMin=[]  ReciprocalOutMax=[]  SumDenOutMin=[]  SumDenOutMax=[]  SumNumOutMin=[]  SumNumOutMax=[]  DivideOutMin=[]  DivideOutMax=[]  UdiffTsProdOutMin=[]  UdiffTsProdOutMax=[]  NTsProdOutMin=[]  NTsProdOutMax=[]  UintegralTsProdOutMin=[]  UintegralTsProdOutMax=[]  UngainTsProdOutMin=[]  UngainTsProdOutMax=[]  IntegratorContinuousStateAttributes=''  IntegratorStateMustResolveToSignalObject=off  IntegratorRTWStateStorageClass=Auto  FilterContinuousStateAttributes=''  FilterStateMustResolveToSignalObject=off  FilterRTWStateStorageClass=Auto  ParallelPVariant=ExternalParameters  IdealPVariant=Disabled  IVariant=ExternalParameters  DVariant=ExternalParameters  IntegratorVariant=Continuous  SatVariant=Disabled  AWVariant=Passthrough  PCopyVariant=Disabled  TRVariant=Disabled  FdbkBlocksVariant=Forward  IdealPFdbkVariant=Disabled  SatFdbkVariant=Disabled  DerivativeFilterVariant=ContFilter  NVariant=ExternalParameters  NCopyVariant=Disabled  FilterICVariant=InternalICsFilter  IntegratorICVariant=InternalICs  ExternalResetVariant=Disabled  TRSumVariant=Passthrough  SumFdbkVariant=Disabled  SumVariant=Sum_PID  TsampFilterVariant=InternalTs  TsampNgainVariant=Passthrough  TsampIntegralVariant=Passthrough  ExternalSaturationOutDataTypeStr=Inherit: Same as second input
  Sum : Sum  Inputs=|+-
  mass : Gain  Gain=mass
  U1* : Outport
  wires:
  Y*/1 -> Sum/1
  Y/1 -> Sum/2
  Add/1 -> U1*/1
  mass/1 -> Add/2
  Sum/1 -> PID Altitude/1
  PID Altitude/1 -> Add/1
  g/1 -> mass/1
  AltPID/1 -> Demux/1
  Demux/1 -> PID Altitude/2
  Demux/2 -> PID Altitude/3
  Demux/3 -> PID Altitude/4
  Constant/1 -> PID Altitude/5

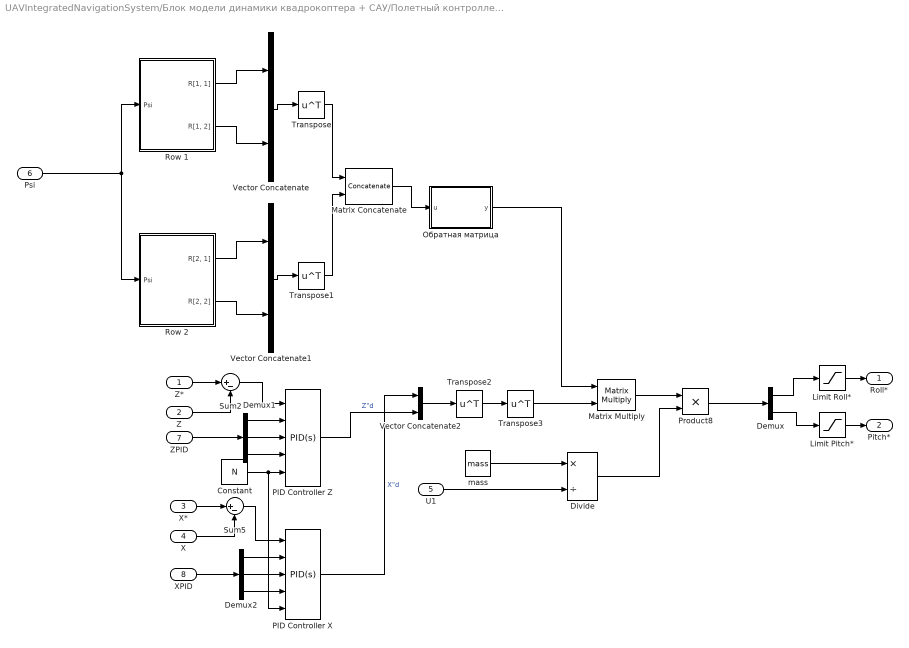
== system UAVIntegratedNavigationSystem/Блок модели динамики квадрокоптера + САУ/Полетный контроллер/Удержание положения ==
  Z* : Inport
  Z : Inport  Port=2
  X* : Inport  Port=3
  X : Inport  Port=4
  U1 : Inport  Port=5
  Psi : Inport  Port=6
  ZPID : Inport  Port=7
  XPID : Inport  Port=8
  Constant : Constant  Value=N
  Demux : Demux  Outputs=2
  Demux1 : Demux  Outputs=3
  Demux2 : Demux  Outputs=3
  Divide : Product  Inputs=*/
  Limit Pitch* : Saturate  UpperLimit=PitchUp  LowerLimit=PitchDown
  Limit Roll* : Saturate  UpperLimit=RollUp  LowerLimit=RollDown
  Matrix Concatenate : Concatenate  Mode=Multidimensional array
  Matrix Multiply : Product  Multiplication=Matrix(*)
  PID Controller X : pid_lib/PID Controller  Controller=PID  Form=Parallel  TimeDomain=Continuous-time  UseExternalTs=off  SampleTime=-1  IntegratorMethod=Forward Euler  FilterMethod=Forward Euler  ControllerParametersSource=external  P=1  I=0  D=0  UseFilter=on  N=100  TunerSelectOption=Transfer Function Based (PID Tuner App)  InitialConditionSource=internal  InitialConditionForIntegrator=0  InitialConditionForFilter=0  DifferentiatorICPrevScaledInput=0  ExternalReset=none  TrackingMode=off  Kt=1  LimitOutput=off  SatLimitsSource=internal  UpperSaturationLimit=inf  LowerSaturationLimit=-inf  LinearizeAsGain=on  AntiWindupMode=none  Kb=1  POutMin=[]  POutMax=[]  IOutMin=[]  IOutMax=[]  DOutMin=[]  DOutMax=[]  NOutMin=[]  NOutMax=[]  SumOutMin=[]  SumOutMax=[]  SaturationOutMin=[]  SaturationOutMax=[]  PParamMin=[]  PParamMax=[]  IParamMin=[]  IParamMax=[]  DParamMin=[]  DParamMax=[]  NParamMin=[]  NParamMax=[]  KbParamMin=[]  KbParamMax=[]  KtParamMin=[]  KtParamMax=[]  KbOutMin=[]  KbOutMax=[]  KtOutMin=[]  KtOutMax=[]  IntegratorOutMin=[]  IntegratorOutMax=[]  FilterOutMin=[]  FilterOutMax=[]  SumI1OutMin=[]  SumI1OutMax=[]  SumI2OutMin=[]  SumI2OutMax=[]  SumI3OutMin=[]  SumI3OutMax=[]  SumI4OutMin=[]  SumI4OutMax=[]  SumDOutMin=[]  SumDOutMax=[]  DifferentiatorOutMin=[]  DifferentiatorOutMax=[]  FilterDiffOutCoefMin=[]  FilterDiffOutCoefMax=[]  ReciprocalOutMin=[]  ReciprocalOutMax=[]  SumDenOutMin=[]  SumDenOutMax=[]  SumNumOutMin=[]  SumNumOutMax=[]  DivideOutMin=[]  DivideOutMax=[]  UdiffTsProdOutMin=[]  UdiffTsProdOutMax=[]  NTsProdOutMin=[]  NTsProdOutMax=[]  UintegralTsProdOutMin=[]  UintegralTsProdOutMax=[]  UngainTsProdOutMin=[]  UngainTsProdOutMax=[]  IntegratorContinuousStateAttributes=''  IntegratorStateMustResolveToSignalObject=off  IntegratorRTWStateStorageClass=Auto  FilterContinuousStateAttributes=''  FilterStateMustResolveToSignalObject=off  FilterRTWStateStorageClass=Auto  ParallelPVariant=ExternalParameters  IdealPVariant=Disabled  IVariant=ExternalParameters  DVariant=ExternalParameters  IntegratorVariant=Continuous  SatVariant=Disabled  AWVariant=Passthrough  PCopyVariant=Disabled  TRVariant=Disabled  FdbkBlocksVariant=Forward  IdealPFdbkVariant=Disabled  SatFdbkVariant=Disabled  DerivativeFilterVariant=ContFilter  NVariant=ExternalParameters  NCopyVariant=Disabled  FilterICVariant=InternalICsFilter  IntegratorICVariant=InternalICs  ExternalResetVariant=Disabled  TRSumVariant=Passthrough  SumFdbkVariant=Disabled  SumVariant=Sum_PID  TsampFilterVariant=InternalTs  TsampNgainVariant=Passthrough  TsampIntegralVariant=Passthrough  ExternalSaturationOutDataTypeStr=Inherit: Same as second input
  PID Controller Z : pid_lib/PID Controller  Controller=PID  Form=Parallel  TimeDomain=Continuous-time  UseExternalTs=off  SampleTime=-1  IntegratorMethod=Forward Euler  FilterMethod=Forward Euler  ControllerParametersSource=external  P=1  I=0  D=0  UseFilter=on  N=100  TunerSelectOption=Transfer Function Based (PID Tuner App)  InitialConditionSource=internal  InitialConditionForIntegrator=0  InitialConditionForFilter=0  DifferentiatorICPrevScaledInput=0  ExternalReset=none  TrackingMode=off  Kt=1  LimitOutput=off  SatLimitsSource=internal  UpperSaturationLimit=inf  LowerSaturationLimit=-inf  LinearizeAsGain=on  AntiWindupMode=none  Kb=1  POutMin=[]  POutMax=[]  IOutMin=[]  IOutMax=[]  DOutMin=[]  DOutMax=[]  NOutMin=[]  NOutMax=[]  SumOutMin=[]  SumOutMax=[]  SaturationOutMin=[]  SaturationOutMax=[]  PParamMin=[]  PParamMax=[]  IParamMin=[]  IParamMax=[]  DParamMin=[]  DParamMax=[]  NParamMin=[]  NParamMax=[]  KbParamMin=[]  KbParamMax=[]  KtParamMin=[]  KtParamMax=[]  KbOutMin=[]  KbOutMax=[]  KtOutMin=[]  KtOutMax=[]  IntegratorOutMin=[]  IntegratorOutMax=[]  FilterOutMin=[]  FilterOutMax=[]  SumI1OutMin=[]  SumI1OutMax=[]  SumI2OutMin=[]  SumI2OutMax=[]  SumI3OutMin=[]  SumI3OutMax=[]  SumI4OutMin=[]  SumI4OutMax=[]  SumDOutMin=[]  SumDOutMax=[]  DifferentiatorOutMin=[]  DifferentiatorOutMax=[]  FilterDiffOutCoefMin=[]  FilterDiffOutCoefMax=[]  ReciprocalOutMin=[]  ReciprocalOutMax=[]  SumDenOutMin=[]  SumDenOutMax=[]  SumNumOutMin=[]  SumNumOutMax=[]  DivideOutMin=[]  DivideOutMax=[]  UdiffTsProdOutMin=[]  UdiffTsProdOutMax=[]  NTsProdOutMin=[]  NTsProdOutMax=[]  UintegralTsProdOutMin=[]  UintegralTsProdOutMax=[]  UngainTsProdOutMin=[]  UngainTsProdOutMax=[]  IntegratorContinuousStateAttributes=''  IntegratorStateMustResolveToSignalObject=off  IntegratorRTWStateStorageClass=Auto  FilterContinuousStateAttributes=''  FilterStateMustResolveToSignalObject=off  FilterRTWStateStorageClass=Auto  ParallelPVariant=ExternalParameters  IdealPVariant=Disabled  IVariant=ExternalParameters  DVariant=ExternalParameters  IntegratorVariant=Continuous  SatVariant=Disabled  AWVariant=Passthrough  PCopyVariant=Disabled  TRVariant=Disabled  FdbkBlocksVariant=Forward  IdealPFdbkVariant=Disabled  SatFdbkVariant=Disabled  DerivativeFilterVariant=ContFilter  NVariant=ExternalParameters  NCopyVariant=Disabled  FilterICVariant=InternalICsFilter  IntegratorICVariant=InternalICs  ExternalResetVariant=Disabled  TRSumVariant=Passthrough  SumFdbkVariant=Disabled  SumVariant=Sum_PID  TsampFilterVariant=InternalTs  TsampNgainVariant=Passthrough  TsampIntegralVariant=Passthrough  ExternalSaturationOutDataTypeStr=Inherit: Same as second input
  Product8 : Product
  Row 1 : Subsystem
  Row 2 : Subsystem
  Sum2 : Sum  Inputs=|+-
  Sum5 : Sum  Inputs=|+-
  Transpose{,1..3} (4 alike) : Math  Operator=transpose  SaturateOnIntegerOverflow=on
  Vector Concatenate : Concatenate
  Vector Concatenate1 : Concatenate
  Vector Concatenate2 : Concatenate
  mass : Constant  Value=mass
  "Обратная матрица " : MATLAB Function  TreatAsAtomicUnit=on
  Roll* : Outport
  Pitch* : Outport  Port=2
  wires:
  Z*/1 -> Sum2/1
  X*/1 -> Sum5/1
  Z/1 -> Sum2/2
  Sum2/1 -> PID Controller Z/1
  Sum5/1 -> PID Controller X/1
  X/1 -> Sum5/2
  U1/1 -> Divide/2
  mass/1 -> Divide/1
  Psi/1 -> Row 1/1(Psi), Row 2/1(Psi)
  PID Controller Z/1 -> Vector Concatenate2/2  "Z\"d"
  Divide/1 -> Product8/2
  PID Controller X/1 -> Vector Concatenate2/1  "X\"d"
  Transpose1/1 -> Matrix Concatenate/2
  Transpose/1 -> Matrix Concatenate/1
  Vector Concatenate/1 -> Transpose/1
  Row 2/2("R[2, 2]") -> Vector Concatenate1/2
  Vector Concatenate1/1 -> Transpose1/1
  Row 1/2("R[1, 2]") -> Vector Concatenate/2
  Row 2/1("R[2, 1]") -> Vector Concatenate1/1
  Row 1/1("R[1, 1]") -> Vector Concatenate/1
  Matrix Concatenate/1 -> "Обратная матрица "/1(u)
  "Обратная матрица "/1(y) -> Matrix Multiply/1
  Vector Concatenate2/1 -> Transpose2/1
  Transpose2/1 -> Transpose3/1
  Transpose3/1 -> Matrix Multiply/2
  Matrix Multiply/1 -> Product8/1
  Product8/1 -> Demux/1
  Demux/2 -> Limit Pitch*/1
  Demux/1 -> Limit Roll*/1
  Limit Roll*/1 -> Roll*/1
  Limit Pitch*/1 -> Pitch*/1
  Constant/1 -> PID Controller X/5, PID Controller Z/5
  ZPID/1 -> Demux1/1
  Demux1/1 -> PID Controller Z/2
  Demux1/2 -> PID Controller Z/3
  Demux1/3 -> PID Controller Z/4
  Demux2/1 -> PID Controller X/2
  Demux2/2 -> PID Controller X/3
  Demux2/3 -> PID Controller X/4
  XPID/1 -> Demux2/1

== system UAVIntegratedNavigationSystem/Блок модели динамики квадрокоптера + САУ/Упрощенная динамика БЛА /Векторы ускорений действующих сил ==
  U1 : Inport
  Pitch : Inport  Port=2
  Roll : Inport  Port=3
  Psi : Inport  Port=4
  g : Inport  Port=5
  "(X, Y, Z, phi)" : Inport  Port=6
  Относительное и Кориолисово ускорение : Inport  Port=7
  Bus Creator : BusCreator  Inputs=4
  Demux : Demux  Outputs=2
  Gain : Gain  Gain=-1
  Ускорение силы гравитации : Subsystem
  Ускорение силы тяги : Subsystem
  "Векторы ускорений, 3 x [3 x 1]" : Outport
  wires:
  Ускорение силы гравитации/1(Вектор ускорения силы гравитации) -> Bus Creator/2  "Вектор ускорения силы гравитации [3 x 1]"
  Ускорение силы тяги/1(Вектор ускорения силы тяги) -> Bus Creator/1  "Вектор ускорения силы тяги [3 x 1]"
  Roll/1 -> Ускорение силы тяги/3(Roll)
  U1/1 -> Ускорение силы тяги/1(U1)
  Pitch/1 -> Ускорение силы тяги/2(Pitch)
  Psi/1 -> Ускорение силы тяги/4(Psi)
  g/1 -> Ускорение силы гравитации/1(g)
  Bus Creator/1 -> "Векторы ускорений, 3 x [3 x 1]"/1
  "(X, Y, Z, phi)"/1 -> Ускорение силы гравитации/2("(X, Y, Z, phi)")
  Относительное и Кориолисово ускорение/1 -> Gain/1
  Demux/1 -> Bus Creator/3  "Вектор относительного ускорения [3 x 1]"
  Gain/1 -> Demux/1
  Demux/2 -> Bus Creator/4  "Вектор Кориолисова ускорения [3 x 1]"

== system UAVIntegratedNavigationSystem/Блок модели динамики квадрокоптера + САУ/Упрощенная динамика БЛА /Моменты управляемых сил ==
  U2 : Inport
  U4 : Inport  Port=2
  U3 : Inport  Port=3
  Mux : Mux  Inputs=3
  "(Mx,My, Mz)" : Outport
  wires:
  U4/1 -> Mux/2
  Mux/1 -> "(Mx,My, Mz)"/1
  U2/1 -> Mux/1
  U3/1 -> Mux/3

== system UAVIntegratedNavigationSystem/Блок модели динамики квадрокоптера + САУ/Упрощенная динамика БЛА /Простр. движение Ц.М. БПЛА (Геогр. СК) ==
  Acc X : Inport
  Acc Y : Inport  Port=2
  AccZ : Inport  Port=3
  "Север(0), Восток(0)" : Inport  Port=4
  Bus Selector : BusSelector  OutputSignals=phi
  Demux1 : Demux  Outputs=3
  Demux2 : Demux  Outputs=2
  Divide : Product  Inputs=*/
  Divide1 : Product  Inputs=*/
  Divide2 : Product  Inputs=*/
  Gain : Gain  Gain=-1
  Mux : Mux  Inputs=3
  Terminator3 : Terminator
  Координаты БПЛА (Географ. СК) : Subsystem
  Радиус - вектор точки местоположения Ц.М. БПЛА (phi) : Subsystem
  Скорости БПЛА (Географ. СК) : Subsystem
  "(X, Y, Z, phi, lambda)" : Outport
  (Vx,Vy,Vz) : Outport  Port=2
  Относительное и Кориолисово ускорение : Outport  Port=3
  Угловая скорость вращения трехгранника : Outport  Port=4
  wires:
  Радиус - вектор точки местоположения Ц.М. БПЛА (phi)/1("R, м") -> Demux2/1, Координаты БПЛА (Географ. СК)/2(R), Скорости БПЛА (Географ. СК)/4(R)
  Скорости БПЛА (Географ. СК)/1(Velocity) -> (Vx,Vy,Vz)/1, Demux1/1, Координаты БПЛА (Географ. СК)/1(Velocity)
  Acc Y/1 -> Скорости БПЛА (Географ. СК)/2(AccY)
  Координаты БПЛА (Географ. СК)/1("Coord, phi, lambda") -> "(X, Y, Z, phi, lambda)"/1, Bus Selector/1
  Acc X/1 -> Скорости БПЛА (Географ. СК)/1(AccX)
  AccZ/1 -> Скорости БПЛА (Географ. СК)/3(AccZ)
  Bus Selector/1 -> Радиус - вектор точки местоположения Ц.М. БПЛА (phi)/1(Phi), Скорости БПЛА (Географ. СК)/5(phi)  "<phi>"
  Скорости БПЛА (Географ. СК)/2(Относ и Кориолис ускорение) -> Относительное и Кориолисово ускорение/1
  Mux/1 -> Угловая скорость вращения трехгранника/1
  Divide/1 -> Mux/1
  Demux1/3 -> Divide1/1, Divide/1
  Demux2/1 -> Divide/2, Divide2/2
  Divide1/1 -> Mux/2
  Demux2/2 -> Divide1/2
  Demux1/2 -> Terminator3/1
  Divide2/1 -> Mux/3
  Demux1/1 -> Gain/1
  Gain/1 -> Divide2/1
  "Север(0), Восток(0)"/1 -> Координаты БПЛА (Географ. СК)/3("Север(0), Восток(0)")

== system UAVIntegratedNavigationSystem/Блок модели динамики квадрокоптера + САУ/Упрощенная динамика БЛА /Решение уравнения Пуассона ==
  AngVelocity : Inport
  Demux : Demux  Outputs=3
  Integrator : Integrator  InitialCondition=[1, 0, 0, 0]
  Mux4 : Mux  Inputs=2
  Quaternions to Rotation Angles : sharedtransform/Quaternions to Rotation Angles  rotationOrder=YZX  aMode=aMode
      settings: SourceProductBaseCode=AE,PW,MT,UV,VE,VP
  ДУ кватернион : Subsystem
  Нормирование кватерниона : Subsystem
  Roll : Outport
  Pitch : Outport  Port=2
  Psi : Outport  Port=3
  wires:
  Integrator/1 -> Нормирование кватерниона/1(q)
  ДУ кватернион/1(d(Q)/dt) -> Integrator/1
  Нормирование кватерниона/1(qnorm) -> Quaternions to Rotation Angles/1, Mux4/2
  Mux4/1 -> ДУ кватернион/1(state)  "Wx Wy Wz  Q0-Q3"
  Quaternions to Rotation Angles/1 -> Demux/1
  Demux/1 -> Psi/1  "Psi"
  Demux/3 -> Roll/1  "Roll"
  Demux/2 -> Pitch/1  "Pitch"
  AngVelocity/1 -> Mux4/1

== system UAVIntegratedNavigationSystem/Показания АИОН + ЛД/Измерения АИОН + ЛД/Вектор случайных аддитивных ошибок в определении высоты местоположения БЛА ==
  "ФФ " : Subsystem
  Вектор измерительных шумов [1x1] : Outport
  wires:
  "ФФ "/1(Случ. погрешность ЛД по высоте) -> Вектор измерительных шумов [1x1]/1

== system UAVIntegratedNavigationSystem/Показания АИОН + ЛД/Измерения АИОН + ЛД/Вектор случайных аддитивных ошибок в определении координат местоположения БЛА ==
  Mux1 : Mux  Inputs=2
  "ФФ " : Subsystem
  Вектор измерительных шумов [2x1] : Outport
  wires:
  Mux1/1 -> Вектор измерительных шумов [2x1]/1
  "ФФ "/1(Случ. погрешность АИОНпо координатам) -> Mux1/2, Mux1/1

== system UAVIntegratedNavigationSystem/Показания приемника ГНСС/Измерения ГНСС/Вектор случайных аддитивных ошибок в определении координат местопложения БЛА ==
  Mux1 : Mux  Inputs=3
  "ФФ " : Subsystem
  ФФ 1 : Subsystem
  Вектор измерительных шумов [3x1] : Outport
  wires:
  Mux1/1 -> Вектор измерительных шумов [3x1]/1
  "ФФ "/1(Случ. погрешность ГНСС по координатам) -> Mux1/3, Mux1/1
  ФФ 1/1(Случ. погрешность ГНСС по высоте) -> Mux1/2

== system UAVIntegratedNavigationSystem/Показания приемника ГНСС/Измерения ГНСС/Вектор случайных аддитивных ошибок в определении ориентации БЛА ==
  Mux1 : Mux  Inputs=3
  "ФФ " : Subsystem
  Вектор измерительных шумов [3x1] : Outport
  wires:
  Mux1/1 -> Вектор измерительных шумов [3x1]/1
  "ФФ "/1(Случ. погрешность ГНСС по углам) -> Mux1/2, Mux1/3, Mux1/1

== system UAVIntegratedNavigationSystem/Показания приемника ГНСС/Измерения ГНСС/Вектор случайных аддитивных ошибок в определении проекций скорости  БЛА ==
  Mux1 : Mux  Inputs=3
  "ФФ " : Subsystem
  ФФ 1 : Subsystem
  Вектор измерительных шумов [3x1] : Outport
  wires:
  "ФФ "/1(Случ. погрешность ГНСС по скоростям) -> Mux1/3, Mux1/1
  Mux1/1 -> Вектор измерительных шумов [3x1]/1
  ФФ 1/1(Случ. погрешность ГНСС по скоростям) -> Mux1/2

== system UAVIntegratedNavigationSystem/Алгоритм ИНС /Алгоритм Навигации/Скорости БПЛА (Географ. СК)/dVx // dt ==
  AccX : Inport
  R : Inport  Port=2
  Vy : Inport  Port=3
  Vz : Inport  Port=4
  Vx : Inport  Port=5
  phi : Inport  Port=6
  AccX Кориолис : Subsystem
  AccX Относительное : Subsystem
  Add : Sum  Inputs=+++
  dVx/dt : Outport
  wires:
  AccX/1 -> Add/1
  Add/1 -> dVx/dt/1
  R/1 -> AccX Относительное/4(R)
  Vx/1 -> AccX Относительное/1(VelX)
  Vy/1 -> AccX Относительное/2(VelY)
  Vz/1 -> AccX Кориолис/1(VelZ), AccX Относительное/3(VelZ)
  phi/1 -> AccX Кориолис/2(phi), AccX Относительное/5(phi)
  AccX Относительное/1(AccX Относительное) -> Add/2
  AccX Кориолис/1(AccX Кориолис) -> Add/3

== system UAVIntegratedNavigationSystem/Алгоритм ИНС /Алгоритм Навигации/Скорости БПЛА (Географ. СК)/dVy // dt ==
  AccY : Inport
  R : Inport  Port=2
  Vz : Inport  Port=3
  Vx : Inport  Port=4
  phi : Inport  Port=5
  AccY Кориолис : Subsystem
  AccY Относительное : Subsystem
  Add : Sum  Inputs=+++
  dVy/dt : Outport
  wires:
  AccY/1 -> Add/1
  Vx/1 -> AccY Относительное/1(VelX)
  R/1 -> AccY Относительное/3(R)
  Add/1 -> dVy/dt/1
  Vz/1 -> AccY Кориолис/1(VelZ), AccY Относительное/2(VelZ)
  phi/1 -> AccY Кориолис/2(phi), AccY Относительное/4(phi)
  AccY Кориолис/1(AccX Кориолис) -> Add/3
  AccY Относительное/1(AccY Относительное) -> Add/2

== system UAVIntegratedNavigationSystem/Алгоритм ИНС /Алгоритм Навигации/Скорости БПЛА (Географ. СК)/dVz // dt ==
  AccZ : Inport
  R : Inport  Port=2
  Vy : Inport  Port=3
  Vz : Inport  Port=4
  Vx : Inport  Port=5
  phi : Inport  Port=6
  AccZ Кориолис : Subsystem
  AccZ Относительное : Subsystem
  Add : Sum  Inputs=+++
  dVz/dt : Outport
  wires:
  AccZ/1 -> Add/1
  Add/1 -> dVz/dt/1
  Vx/1 -> AccZ Относительное/1(VelX), AccZ Кориолис/1(VelX)
  Vy/1 -> AccZ Относительное/2(VelY), AccZ Кориолис/2(VelY)
  Vz/1 -> AccZ Относительное/3(VelZ)
  R/1 -> AccZ Относительное/4(R)
  phi/1 -> AccZ Кориолис/3(phi), AccZ Относительное/5(phi)
  AccZ Кориолис/1(AccZ Кориолис) -> Add/3
  AccZ Относительное/1(AccZ Относительное) -> Add/2

== system UAVIntegratedNavigationSystem/Алгоритм ИНС (коррекия БЧЭ)/Алгоритм Навигации/Скорости БПЛА (Географ. СК)/dVx // dt ==
  AccX : Inport
  R : Inport  Port=2
  Vy : Inport  Port=3
  Vz : Inport  Port=4
  Vx : Inport  Port=5
  phi : Inport  Port=6
  AccX Кориолис : Subsystem
  AccX Относительное : Subsystem
  Add : Sum  Inputs=+++
  dVx/dt : Outport
  wires:
  AccX/1 -> Add/1
  Add/1 -> dVx/dt/1
  R/1 -> AccX Относительное/4(R)
  Vx/1 -> AccX Относительное/1(VelX)
  Vy/1 -> AccX Относительное/2(VelY)
  Vz/1 -> AccX Кориолис/1(VelZ), AccX Относительное/3(VelZ)
  phi/1 -> AccX Кориолис/2(phi), AccX Относительное/5(phi)
  AccX Относительное/1(AccX Относительное) -> Add/2
  AccX Кориолис/1(AccX Кориолис) -> Add/3

== system UAVIntegratedNavigationSystem/Алгоритм ИНС (коррекия БЧЭ)/Алгоритм Навигации/Скорости БПЛА (Географ. СК)/dVy // dt ==
  AccY : Inport
  R : Inport  Port=2
  Vz : Inport  Port=3
  Vx : Inport  Port=4
  phi : Inport  Port=5
  AccY Кориолис : Subsystem
  AccY Относительное : Subsystem
  Add : Sum  Inputs=+++
  dVy/dt : Outport
  wires:
  AccY/1 -> Add/1
  Vx/1 -> AccY Относительное/1(VelX)
  R/1 -> AccY Относительное/3(R)
  Add/1 -> dVy/dt/1
  Vz/1 -> AccY Кориолис/1(VelZ), AccY Относительное/2(VelZ)
  phi/1 -> AccY Кориолис/2(phi), AccY Относительное/4(phi)
  AccY Кориолис/1(AccX Кориолис) -> Add/3
  AccY Относительное/1(AccY Относительное) -> Add/2

== system UAVIntegratedNavigationSystem/Алгоритм ИНС (коррекия БЧЭ)/Алгоритм Навигации/Скорости БПЛА (Географ. СК)/dVz // dt ==
  AccZ : Inport
  R : Inport  Port=2
  Vy : Inport  Port=3
  Vz : Inport  Port=4
  Vx : Inport  Port=5
  phi : Inport  Port=6
  AccZ Кориолис : Subsystem
  AccZ Относительное : Subsystem
  Add : Sum  Inputs=+++
  dVz/dt : Outport
  wires:
  AccZ/1 -> Add/1
  Add/1 -> dVz/dt/1
  Vx/1 -> AccZ Относительное/1(VelX), AccZ Кориолис/1(VelX)
  Vy/1 -> AccZ Относительное/2(VelY), AccZ Кориолис/2(VelY)
  Vz/1 -> AccZ Относительное/3(VelZ)
  R/1 -> AccZ Относительное/4(R)
  phi/1 -> AccZ Кориолис/3(phi), AccZ Относительное/5(phi)
  AccZ Кориолис/1(AccZ Кориолис) -> Add/3
  AccZ Относительное/1(AccZ Относительное) -> Add/2
